simulink model "plan_a_full_model"  (R2026a)
settings: Solver=FixedStepDiscrete  FixedStep=0.05
settings Model: Creator=rayyan  LastModifiedBy=rayyan

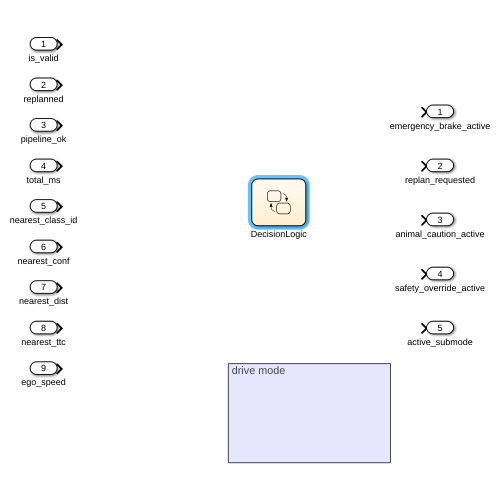
[thumbnail: Simulink's stored preview of the top-level diagram]
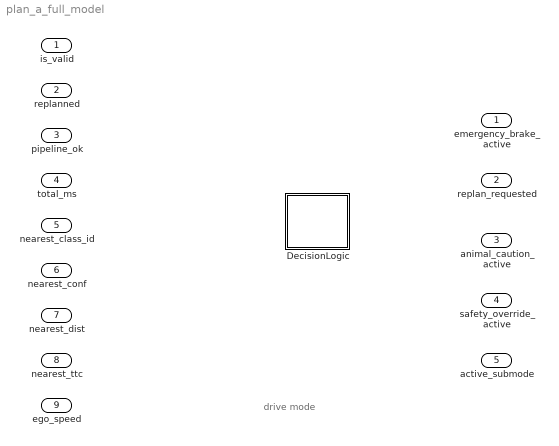
== system plan_a_full_model ==
  note: drive mode
  is_valid : Inport  OutDataTypeStr=boolean
  replanned : Inport  Port=2  OutDataTypeStr=boolean
  pipeline_ok : Inport  Port=3  OutDataTypeStr=boolean
  total_ms : Inport  Port=4  OutDataTypeStr=double
  nearest_class_id : Inport  Port=5  OutDataTypeStr=int32
  nearest_conf : Inport  Port=6  OutDataTypeStr=double
  nearest_dist : Inport  Port=7  OutDataTypeStr=double
  nearest_ttc : Inport  Port=8  OutDataTypeStr=double
  ego_speed : Inport  Port=9  OutDataTypeStr=double
  DecisionLogic : Stateflow chart  TreatAsAtomicUnit=on
  emergency_brake_active : Outport  OutDataTypeStr=boolean
  replan_requested : Outport  Port=2  OutDataTypeStr=boolean
  animal_caution_active : Outport  Port=3  OutDataTypeStr=boolean
  safety_override_active : Outport  Port=4  OutDataTypeStr=boolean
  active_submode : Outport  Port=5  OutDataTypeStr=int32

== stateflow chart plan_a_full_model/DecisionLogic ==
